simulink model "Simulation_GFM"  (R2022b)
settings: Solver=FixedStepAuto  StartTime=0.0  StopTime=4  FixedStep=1e-6  RelTol=1e-3
model workspace (MAT data in the model file):
  Fbase = 50
  Filter_Ind = 0.00435
  Fs = 10000
  Series1_L = 0.004
  Series2_L = 0.00035
  Shunt_C = 2.2e-06
  Snubber_C = inf
  Snubber_R = 100000
  Test_Interval = 3
  Ts = 0.0001
  VDCref = 48
undefined symbols (not defined in the file): DiscIntNeverNeededParam, Rdamp, Series1_C, Series2_R
libraries: spsThreePhaseSeriesRLCBranchLib x7, spsPWMGeneratorDCDCLib x3, spsVoltageMeasurementLib x3, spsabctodq0Lib x2, spsDCVoltageSourceLib x1, spsThreePhaseVIMeasurementLib x1, spsdq0toabcLib x1, spsUniversalBridgeLib x1, spspowerguiLib x1
settings Model: NumberOfSteps=10000  SnapshotBufferSize=10000  SnapshotInterval=10000  Creator=yanni  LastModifiedBy=yanni

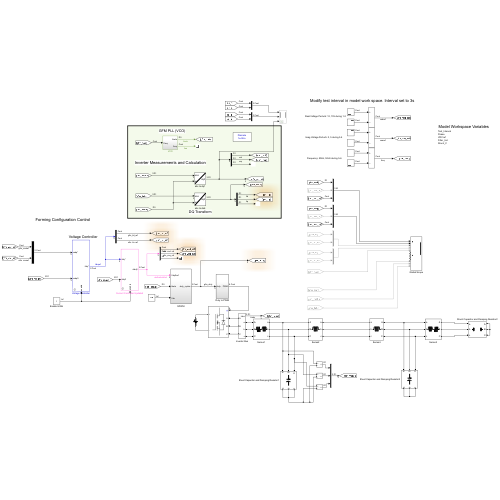
[thumbnail: Simulink's stored preview of the top-level diagram]
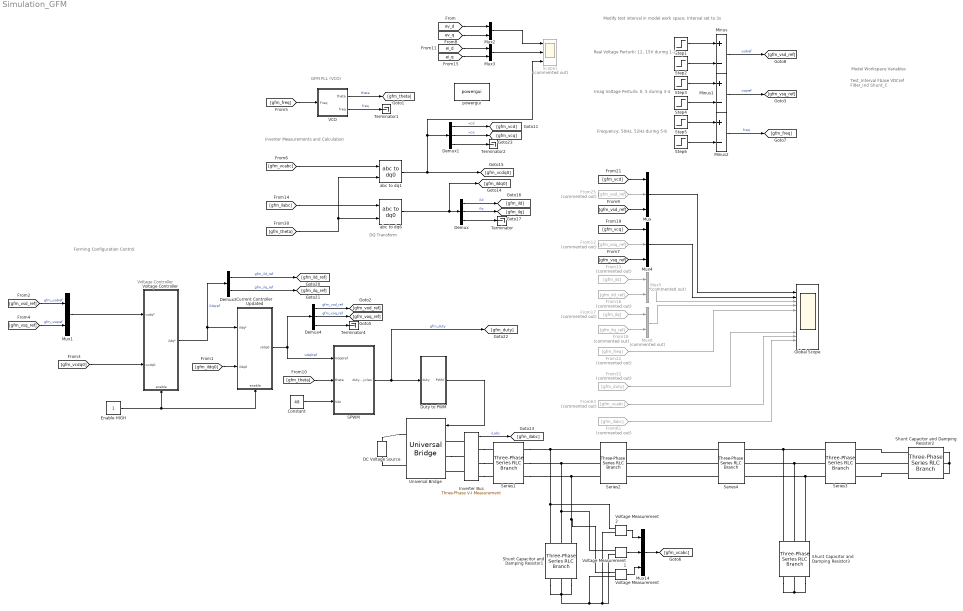
== system Simulation_GFM ==
  note: DQ Transform
  note: Forming Configuration Control
  note: Inverter Measurements and Calculation
  note: Voltage Controller
  note: Model Workspace Variables
  note: Real Voltage Perturb: 12, 15V during 1-2
  note: Imag Voltage Perturb: 0, 5 during 3-4
  note: Frequency: 50Hz, 52Hz during 5-6
  note: Test_Interval
      | Fbase
      | VDCref
      | Filter_Ind
      | Shunt_C
  note: Modify test interval in model work space. Interval set to 3s
  note: GFM PLL (VCO)
  Constant : Constant  Value=48
  Current Controller Updated : Subsystem  mask{Id_Proportional=1.22, Id_Integral=957}
      mask prompts: Id_Proportional "Kp"; Id_Integral "Ki"
      settings: PortSchema="{\"entries\":[{\"content\":{\"sides\":[{\"content\":{\"connectorIds\":[\"In1\",\"In2\"]},\"type\":\"ConnectorPlacement.EquallySpacedRectSide\",\"uuid\":\"134caf41-c34b-48d0-a71a-522329c40d8c\"},{\"content\":{\"connectorIds\":[\"Out1\"],\"side\":\"RIGHT\"},\"type\":\"ConnectorPlacement.EquallySpacedRectSide\",\"uuid\":\"de6d8359-09d9-4cb7-8990-bc4b6d48f18d\"},{\"content\":{\"connectorIds\":[],\"side\":\"TOP\"},\"type\":\"ConnectorPlacement.EquallySpacedRectSide\",\"uuid\":\"e2785d07-2ead-4d42-94ac-8025f550e46a\"},{\"content\":{\"connectorIds\":[\"In3\"],\"side\":\"BOTTOM\"},\"type\":\"ConnectorPlacement.EquallySpacedRectSide\",\"uuid\":\"a912a274-012c-4cba-911c-beb79bb7dc91\"}]},\"type\":\"ConnectorPlacement.EquallySpacedConnector\",\"uuid\":\"3c498838-bb9a-4b09-bf48-00f71cabf7b4\"}],\"packageUris\":[\"http://schema.mathworks.com/mf0/Connector/R2020b\"],\"version\":\"1.0\"}"
  DC Voltage Source : spsDCVoltageSourceLib/DC Voltage Source  Amplitude=48  Measurements=None
  Demux : Demux  Outputs=3
  Demux1 : Demux  Outputs=3
  Demux3 : Demux  Outputs=2
  Demux4 : Demux  Outputs=3
  Duty to PWM : Subsystem
  Enable HIGH : Constant
  From12 : From  Commented=on  GotoTag=gfm_voq_ref
      settings: CloseFcn=tagdialog Close
  From13 : From  Commented=on  GotoTag=gfm_ild
      settings: CloseFcn=tagdialog Close
  From16 : From  Commented=on  GotoTag=gfm_ild_ref
      settings: CloseFcn=tagdialog Close
  From17 : From  Commented=on  GotoTag=gfm_ilq
      settings: CloseFcn=tagdialog Close
  From18 : From  Commented=on  GotoTag=gfm_ilq_ref
      settings: CloseFcn=tagdialog Close
  From22 : From  Commented=on  GotoTag=gfm_freq
  From25 : From  Commented=on  GotoTag=gfm_vod_ref
      settings: CloseFcn=tagdialog Close
  From32 : From  Commented=on  GotoTag=gfm_duty
      settings: CloseFcn=tagdialog Close
  From61 : From  Commented=on  GotoTag=gfm_ilabc
      settings: CloseFcn=tagdialog Close
  From63 : From  Commented=on  GotoTag=gfm_vcabc
      settings: CloseFcn=tagdialog Close
  Global Scope : Scope  NumInputPorts=12
  Inverter Bus : spsThreePhaseVIMeasurementLib/Three-Phase V-I Measurement  VoltageMeasurement=no  SetLabelV=off  LabelV=Vabc  Vpu=off  VpuLL=off  CurrentMeasurement=yes  SetLabelI=off  LabelI=Iabc  Ipu=off  Pbase=100e6  Vbase=500e3  OutputType=Complex  PhasorSimulation=off  PSBequivalent=0
  Minus : Sum  Inputs=+-
  Minus1 : Sum  Inputs=+-
  Minus2 : Sum  Inputs=+-
  Mux : Mux  Inputs=3
  Mux1 : Mux  Inputs=2
  Mux14 : Mux  Inputs=3
  Mux2 : Mux  Inputs=2
  Mux3 : Mux  Inputs=2
  Mux4 : Mux  Inputs=3
  Mux5 : Mux  Commented=on  Inputs=2
  Mux6 : Mux  Commented=on  Inputs=2
  SPWM : Subsystem
  Scope1 : Scope  Commented=on  NumInputPorts=3
  Series1 : spsThreePhaseSeriesRLCBranchLib/Three-Phase Series RLC Branch  LConnTagsString=A|B|C  RConnTagsString=A|B|C  BranchType=RL  Resistance=0.35  Inductance=Series1_L  Capacitance=Series1_C  Measurements=None
  Series2 : spsThreePhaseSeriesRLCBranchLib/Three-Phase Series RLC Branch  LConnTagsString=A|B|C  RConnTagsString=A|B|C  BranchType=L  Resistance=Series2_R  Inductance=Series2_L  Capacitance=1e-6  Measurements=None
  Series3 : spsThreePhaseSeriesRLCBranchLib/Three-Phase Series RLC Branch  LConnTagsString=A|B|C  RConnTagsString=A|B|C  BranchType=RL  Resistance=0.35  Inductance=Series1_L  Capacitance=Series1_C  Measurements=None
  Series4 : spsThreePhaseSeriesRLCBranchLib/Three-Phase Series RLC Branch  LConnTagsString=A|B|C  RConnTagsString=A|B|C  BranchType=L  Resistance=Series2_L  Inductance=Series2_L  Capacitance=1e-6  Measurements=None
  Shunt Capacitor and Damping Resistor1 : spsThreePhaseSeriesRLCBranchLib/Three-Phase Series RLC Branch  LConnTagsString=A|B|C  RConnTagsString=A|B|C  BranchType=C  Resistance=Rdamp  Inductance=1e-3  Capacitance=2.2e-6  Measurements=None
  Shunt Capacitor and Damping Resistor2 : spsThreePhaseSeriesRLCBranchLib/Three-Phase Series RLC Branch  LConnTagsString=A|B|C  RConnTagsString=A|B|C  BranchType=Open circuit  Resistance=20  Inductance=1e-3  Capacitance=Shunt_C  Measurements=None
  Shunt Capacitor and Damping Resistor3 : spsThreePhaseSeriesRLCBranchLib/Three-Phase Series RLC Branch  LConnTagsString=A|B|C  RConnTagsString=A|B|C  BranchType=C  Resistance=Rdamp  Inductance=1e-3  Capacitance=2.2e-6  Measurements=None
  Step1 : Step  Time=Test_Interval*1  Before=12  After=15
  Step2 : Step  Time=Test_Interval*2  After=3
  Step3 : Step  Time=Test_Interval*3  After=5
  Step4 : Step  Time=Test_Interval*4  After=5
  Step5 : Step  Time=Test_Interval*5  Before=50  After=52  SampleTime=0
  Step6 : Step  Time=Test_Interval*6  After=2
  Terminator{,1..2,4} (4 alike) : Terminator
  Universal Bridge : spsUniversalBridgeLib/Universal Bridge  Arms=3  SnubberResistance=Snubber_R  SnubberCapacitance=Snubber_C  Device=MOSFET / Diodes  Ron=1e-3  Lon=0  ForwardVoltages="[  0  0  ]"  ForwardVoltage=0  GTOparameters=[ 10e-6 , 20e-6 ]  IGBTparameters=[ 1e-6 , 2e-6 ]  Measurements=None  Measurements_2=None  converterType=Rectifier
  VCO : Subsystem
  Voltage Controller : Subsystem  mask{Id_Proportional=0.028, Id_Integral=8.8685}
      mask prompts: Id_Proportional "Kp"; Id_Integral "Ki"
      settings: PortSchema="{\"entries\":[{\"content\":{\"sides\":[{\"content\":{\"connectorIds\":[\"In1\",\"In2\"]},\"type\":\"ConnectorPlacement.EquallySpacedRectSide\",\"uuid\":\"134caf41-c34b-48d0-a71a-522329c40d8c\"},{\"content\":{\"connectorIds\":[\"Out1\"],\"side\":\"RIGHT\"},\"type\":\"ConnectorPlacement.EquallySpacedRectSide\",\"uuid\":\"de6d8359-09d9-4cb7-8990-bc4b6d48f18d\"},{\"content\":{\"connectorIds\":[],\"side\":\"TOP\"},\"type\":\"ConnectorPlacement.EquallySpacedRectSide\",\"uuid\":\"e2785d07-2ead-4d42-94ac-8025f550e46a\"},{\"content\":{\"connectorIds\":[\"In3\"],\"side\":\"BOTTOM\"},\"type\":\"ConnectorPlacement.EquallySpacedRectSide\",\"uuid\":\"a912a274-012c-4cba-911c-beb79bb7dc91\"}]},\"type\":\"ConnectorPlacement.EquallySpacedConnector\",\"uuid\":\"3c498838-bb9a-4b09-bf48-00f71cabf7b4\"}],\"packageUris\":[\"http://schema.mathworks.com/mf0/Connector/R2020b\"],\"version\":\"1.0\"}"
  Voltage Measurement : spsVoltageMeasurementLib/Voltage Measurement  PhasorSimulation=off  OutputType=Complex  PSBequivalent=0
  Voltage Measurement1 : spsVoltageMeasurementLib/Voltage Measurement  PhasorSimulation=off  OutputType=Complex  PSBequivalent=0
  Voltage Measurement2 : spsVoltageMeasurementLib/Voltage Measurement  PhasorSimulation=off  OutputType=Complex  PSBequivalent=0
  abc to dq1 : spsabctodq0Lib/abc to dq0  Alignment=90 degrees behind phase A axis
  abc to dq6 : spsabctodq0Lib/abc to dq0  Alignment=90 degrees behind phase A axis
  powergui : spspowerguiLib/powergui  Priority=1  SimulationMode=Discrete  SampleTime=1e-6  frequency=60  Iterations=50  frequencyindice=0  Pbase=100e6  ErrMax=1e-4  UnitsV=kV  UnitsW=MW  buscounter=0  FunctionMessages=off  echomessages=off  EnableUseOfTLC=off  CurrentSourceSwitches=off  DisableSnubberDevices=off  DisableRonSwitches=off  DisableVfSwitches=off  DisplayEquations=off  AutomaticDiscreteSolvers=off  SolverType=Tustin/Backward Euler (TBE)  Interpol=off  ExternalGateDelay=off  methode=off  Ts=100  x0status=blocks  SPID=on  SwTol=0  HookPort=off  NonlinearTolerance=1e-4  nMaxIteration=100  ContinueOnMaxIteration=off  RestoreLinks=warning  ResistiveCurrentMeasurement=off  Frange=[0:2:500]  Ylog=off  Xlog=on  ShowGrid=off  save=off  variable=ZData  structure=0  ZoomFFT=off  StartTime=0.0  cycles=1  DisplayStyle=1  fundamental=60  FreqAxis=off  MaxFrequency=1000  frequencyindicesteady=1  RmsSteady=1  display=off
  wires:
  abc to dq1/1 -> Demux1/1, Scope1/3, [gfm_vcdq0]
  Current Controller Updated/1(vtdq0) -> SPWM/1(Vdq0ref), Demux4/1  "vdq0ref"
  abc to dq6/1 -> [gfm_ildq0], Demux/1
  [gfm_theta] -> SPWM/2(theta)
  Enable HIGH/1 -> Current Controller Updated/3(enable), Voltage Controller/3(enable)
  Mux1/1 -> Voltage Controller/1(vsdq*)
  Inverter Bus/1 -> [gfm_ilabc]  "iLabc"
  Demux/2 -> [gfm_ilq]  "ilq"
  Demux/1 -> [gfm_ild]  "ild"
  Demux/3 -> Terminator/1
  Demux3/2 -> [gfm_ilq_ref]  "gfm_ilq_ref"
  Demux3/1 -> [gfm_ild_ref]  "gfm_ild_ref"
  Demux4/2 -> [gfm_voq_ref]  "gfm_voq_ref"
  Demux4/1 -> [gfm_vod_ref]  "gfm_vod_ref"
  Demux4/3 -> Terminator4/1
  [gfm_theta] -> abc to dq1/2, abc to dq6/2
  Voltage Controller/1(ildq*) -> Demux3/1, Current Controller Updated/1(ildq*)  "ildqref"
  [gfm_ilabc] -> abc to dq6/1
  Duty to PWM/1(PWM) -> Universal Bridge/1
  SPWM/1(duty_cycles) -> Duty to PWM/1(duty), [gfm_duty]  "gfm_duty"
  From25/1 -> Mux/2
  From17/1 -> Mux6/1
  Mux/1 -> Global Scope/1
  From63/1 -> Global Scope/11
  From32/1 -> Global Scope/10
  From12/1 -> Mux4/2
  Mux4/1 -> Global Scope/2
  [gfm_vcd] -> Mux/1
  Mux5/1 -> Global Scope/3
  From61/1 -> Global Scope/12
  Mux6/1 -> Global Scope/4
  From16/1 -> Mux5/2
  From13/1 -> Mux5/1
  From18/1 -> Mux6/2
  [gfm_vcq] -> Mux4/1
  [gfm_vsd_ref] -> Mux/3
  [gfm_vsq_ref] -> Mux4/3
  Demux1/2 -> [gfm_vcq]  "vcq"
  Demux1/1 -> [gfm_vcd]  "vcd"
  Demux1/3 -> Terminator2/1
  [gfm_vcabc] -> abc to dq1/1
  [gfm_vcdq0] -> Voltage Controller/2(vcdq0)
  Constant/1 -> SPWM/3(Vdc)
  Minus/1 -> [gfm_vsd_ref]  "vsdref"
  Step3/1 -> Minus1/1
  Step2/1 -> Minus/2
  Minus1/1 -> [gfm_vsq_ref]  "vsqref"
  Step5/1 -> Minus2/1
  Step4/1 -> Minus1/2
  Step1/1 -> Minus/1
  Minus2/1 -> [gfm_freq]  "freq"
  Step6/1 -> Minus2/2
  From22/1 -> Global Scope/5
  [gfm_ildq0] -> Current Controller Updated/2(ildq0)
  [gfm_vsd_ref] -> Mux1/1  "gfm_vsdref"
  [gfm_vsq_ref] -> Mux1/2  "gfm_vsqref"
  VCO/1(theta) -> [gfm_theta]  "theta"
  VCO/2(freq) -> Terminator1/1  "freq"
  [gfm_freq] -> VCO/1(Freq)
  Mux14/1 -> [gfm_vcabc]
  Voltage Measurement/1 -> Mux14/3
  Voltage Measurement1/1 -> Mux14/2
  Voltage Measurement2/1 -> Mux14/1
  Mux3/1 -> Scope1/2
  Mux2/1 -> Scope1/1
  [ev_d] -> Mux2/1
  [ev_q] -> Mux2/2
  [ei_d] -> Mux3/1
  [ei_q] -> Mux3/2
  connections:
  DC Voltage Source/LConn1 -- Universal Bridge/RConn2
  Universal Bridge/RConn1 -- DC Voltage Source/RConn1
  Shunt Capacitor and Damping Resistor1/LConn2 -- Series2/LConn2 -- Series1/RConn2 -- Voltage Measurement1/LConn1
  Voltage Measurement/LConn1 -- Series2/LConn3 -- Series1/RConn3 -- Shunt Capacitor and Damping Resistor1/LConn3
  Voltage Measurement2/LConn1 -- Series2/LConn1 -- Series1/RConn1 -- Shunt Capacitor and Damping Resistor1/LConn1
  Inverter Bus/RConn2 -- Series1/LConn2
  Inverter Bus/RConn1 -- Series1/LConn1
  Inverter Bus/RConn3 -- Series1/LConn3
  Inverter Bus/LConn1 -- Universal Bridge/LConn1
  Universal Bridge/LConn2 -- Inverter Bus/LConn2
  Inverter Bus/LConn3 -- Universal Bridge/LConn3
  Shunt Capacitor and Damping Resistor2/LConn1 -- Shunt Capacitor and Damping Resistor2/LConn2 -- Shunt Capacitor and Damping Resistor2/LConn3
  Shunt Capacitor and Damping Resistor1/RConn2 -- Voltage Measurement/LConn2 -- Voltage Measurement2/LConn2 -- Voltage Measurement1/LConn2 -- Shunt Capacitor and Damping Resistor1/RConn1 -- Shunt Capacitor and Damping Resistor1/RConn3
  Shunt Capacitor and Damping Resistor3/RConn2 -- Shunt Capacitor and Damping Resistor3/RConn3 -- Shunt Capacitor and Damping Resistor3/RConn1
  Shunt Capacitor and Damping Resistor3/LConn2 -- Series3/RConn2 -- Series4/LConn2
  Shunt Capacitor and Damping Resistor3/LConn3 -- Series3/RConn3 -- Series4/LConn3
  Shunt Capacitor and Damping Resistor3/LConn1 -- Series3/RConn1 -- Series4/LConn1
  Shunt Capacitor and Damping Resistor2/RConn1 -- Series3/LConn1
  Shunt Capacitor and Damping Resistor2/RConn3 -- Series3/LConn3
  Shunt Capacitor and Damping Resistor2/RConn2 -- Series3/LConn2
  Series4/RConn1 -- Series2/RConn1
  Series4/RConn2 -- Series2/RConn2
  Series4/RConn3 -- Series2/RConn3

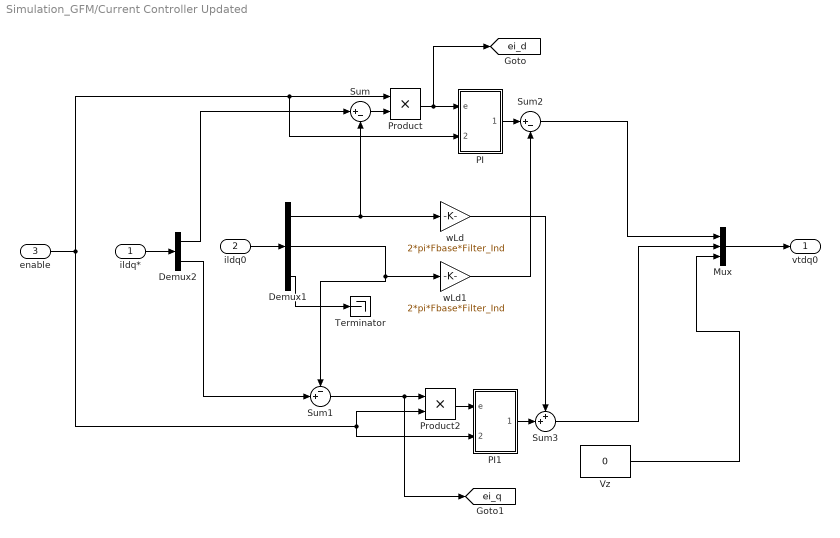
== system Simulation_GFM/Current Controller Updated ==
  ildq* : Inport
  ildq0 : Inport  Port=2
  enable : Inport  Port=3
  Demux1 : Demux  Outputs=3
  Demux2 : Demux  Outputs=2
  Mux : Mux  Inputs=3
  PI : Subsystem
  PI1 : Subsystem
  Product : Product  RndMeth=Zero
  Product2 : Product  RndMeth=Zero
  Sum : Sum  Inputs=|+-
  Sum1 : Sum  Inputs=-+|
  Sum2 : Sum  Inputs=|+-
  Sum3 : Sum  Inputs=++|
  Terminator : Terminator
  Vz : Constant  Value=0
  wLd : Gain  Gain=2*pi*Fbase*Filter_Ind
  wLd1 : Gain  Gain=2*pi*Fbase*Filter_Ind
  vtdq0 : Outport
  tag scope: ei_d=global, ei_q=global
  wires:
  Sum2/1 -> Mux/1
  Sum3/1 -> Mux/2
  ildq0/1 -> Demux1/1
  Mux/1 -> vtdq0/1
  Demux1/3 -> Terminator/1
  ildq*/1 -> Demux2/1
  Demux2/1 -> Sum/1
  Demux2/2 -> Sum1/2
  PI/1(Out) -> Sum2/1
  wLd/1 -> Sum3/1
  wLd1/1 -> Sum2/2
  PI1/1(Out) -> Sum3/2
  Demux1/2 -> Sum1/1, wLd1/1
  Demux1/1 -> wLd/1, Sum/2
  Product2/1 -> PI1/1(e)
  Sum/1 -> Product/2
  enable/1 -> Product/1, PI/2(RST), PI1/2(RST), Product2/2
  Vz/1 -> Mux/3
  Sum1/1 -> [ei_q], Product2/1
  Product/1 -> [ei_d], PI/1(e)

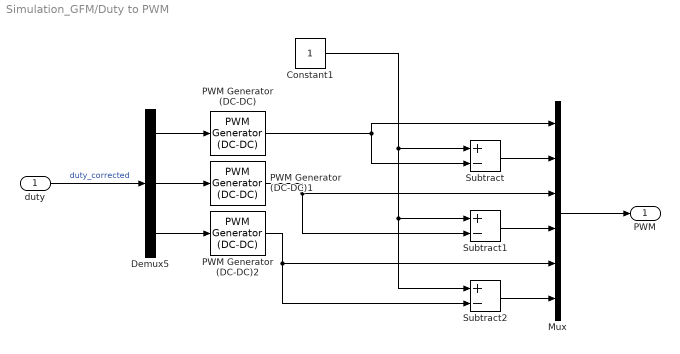
== system Simulation_GFM/Duty to PWM ==
  duty : Inport
  Constant1 : Constant
  Demux5 : Demux  Outputs=3
  Mux : Mux  Inputs=6
  PWM Generator (DC-DC) : spsPWMGeneratorDCDCLib/PWM Generator (DC-DC)  Fsw=Fs  Ts=0
  PWM Generator (DC-DC)1 : spsPWMGeneratorDCDCLib/PWM Generator (DC-DC)  Fsw=Fs  Ts=0
  PWM Generator (DC-DC)2 : spsPWMGeneratorDCDCLib/PWM Generator (DC-DC)  Fsw=Fs  Ts=0
  Subtract : Sum  Inputs=+-
  Subtract1 : Sum  Inputs=+-
  Subtract2 : Sum  Inputs=+-
  PWM : Outport
  wires:
  PWM Generator (DC-DC)1/1 -> Subtract1/2, Mux/3
  Demux5/2 -> PWM Generator (DC-DC)1/1
  Demux5/1 -> PWM Generator (DC-DC)/1
  Demux5/3 -> PWM Generator (DC-DC)2/1
  PWM Generator (DC-DC)2/1 -> Subtract2/2, Mux/5
  duty/1 -> Demux5/1  "duty_corrected"
  Subtract1/1 -> Mux/4
  Subtract2/1 -> Mux/6
  PWM Generator (DC-DC)/1 -> Mux/1, Subtract/2
  Constant1/1 -> Subtract2/1, Subtract1/1, Subtract/1
  Subtract/1 -> Mux/2
  Mux/1 -> PWM/1

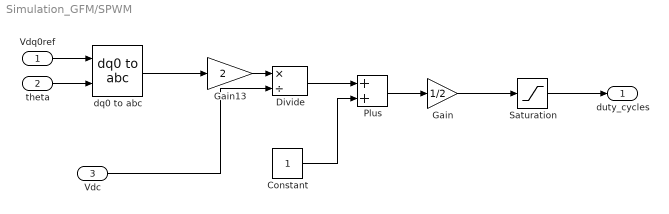
== system Simulation_GFM/SPWM ==
  Vdq0ref : Inport
  theta : Inport  Port=2
  Vdc : Inport  Port=3
  Constant : Constant
  Divide : Product  Inputs=*/
  Gain : Gain  Gain=1/2
  Gain13 : Gain  Gain=2
  Plus : Sum
  Saturation : Saturate  UpperLimit=0.9  LowerLimit=0.1
  dq0 to abc : spsdq0toabcLib/dq0 to abc  Alignment=90 degrees behind phase A axis
  duty_cycles : Outport
  wires:
  Vdq0ref/1 -> dq0 to abc/1
  Gain/1 -> Saturation/1
  theta/1 -> dq0 to abc/2
  Constant/1 -> Plus/2
  Plus/1 -> Gain/1
  Saturation/1 -> duty_cycles/1
  dq0 to abc/1 -> Gain13/1
  Gain13/1 -> Divide/1
  Vdc/1 -> Divide/2
  Divide/1 -> Plus/1

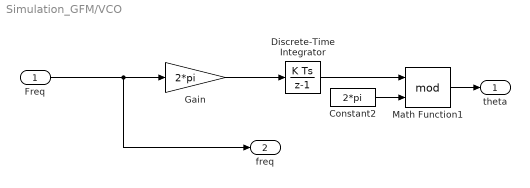
== system Simulation_GFM/VCO ==
  Freq : Inport
  Constant2 : Constant  Value=2*pi
  Discrete-Time Integrator : DiscreteIntegrator  SampleTime=Ts  ICPrevOutput=DiscIntNeverNeededParam  ICPrevScaledInput=DiscIntNeverNeededParam
  Gain : Gain  Gain=2*pi
  Math Function1 : Math  Operator=mod  SignedPower=on
  theta : Outport
  freq : Outport  Port=2
  wires:
  Constant2/1 -> Math Function1/2
  Discrete-Time Integrator/1 -> Math Function1/1
  Math Function1/1 -> theta/1
  Freq/1 -> Gain/1, freq/1
  Gain/1 -> Discrete-Time Integrator/1

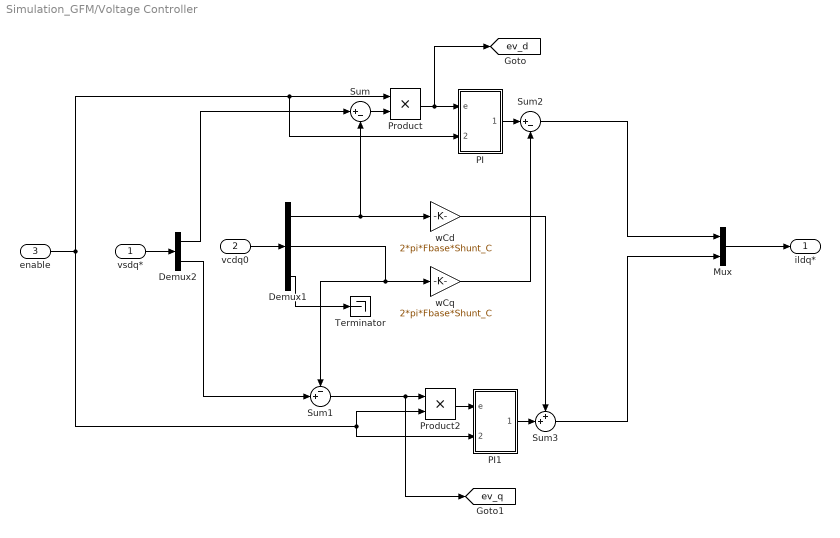
== system Simulation_GFM/Voltage Controller ==
  vsdq* : Inport
  vcdq0 : Inport  Port=2
  enable : Inport  Port=3
  Demux1 : Demux  Outputs=3
  Demux2 : Demux  Outputs=2
  Mux : Mux  Inputs=2
  PI : Subsystem
  PI1 : Subsystem
  Product : Product  RndMeth=Zero
  Product2 : Product  RndMeth=Zero
  Sum : Sum  Inputs=|+-
  Sum1 : Sum  Inputs=-+|
  Sum2 : Sum  Inputs=|+-
  Sum3 : Sum  Inputs=++|
  Terminator : Terminator
  wCd : Gain  Gain=2*pi*Fbase*Shunt_C
  wCq : Gain  Gain=2*pi*Fbase*Shunt_C
  ildq* : Outport
  tag scope: ev_d=global, ev_q=global
  wires:
  Sum2/1 -> Mux/1
  Sum3/1 -> Mux/2
  vcdq0/1 -> Demux1/1
  Mux/1 -> ildq*/1
  Demux1/3 -> Terminator/1
  vsdq*/1 -> Demux2/1
  Demux2/1 -> Sum/1
  Demux2/2 -> Sum1/2
  Product/1 -> [ev_d], PI/1(e)
  Sum1/1 -> [ev_q], Product2/1
  PI/1(Out) -> Sum2/1
  wCd/1 -> Sum3/1
  wCq/1 -> Sum2/2
  PI1/1(Out) -> Sum3/2
  Demux1/2 -> Sum1/1, wCq/1
  Demux1/1 -> wCd/1, Sum/2
  Product2/1 -> PI1/1(e)
  Sum/1 -> Product/2
  enable/1 -> Product/1, PI/2(RST), PI1/2(RST), Product2/2

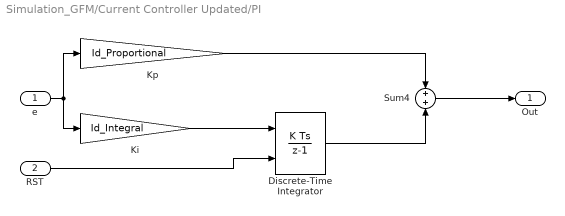
== system Simulation_GFM/Current Controller Updated/PI ==
  e : Inport
  RST : Inport  Port=2
  Discrete-Time Integrator : DiscreteIntegrator  gainval=1  ExternalReset=either  SampleTime=Ts  LimitOutput=on  UpperSaturationLimit=20000  LowerSaturationLimit=-20000  ICPrevOutput=DiscIntNeverNeededParam  ICPrevScaledInput=DiscIntNeverNeededParam
  Ki : Gain  Gain=Id_Integral  SaturateOnIntegerOverflow=on  OutDataTypeStr=Inherit: Same as input  ParamDataTypeStr=Inherit: Same as input
  Kp : Gain  Gain=Id_Proportional  SaturateOnIntegerOverflow=on  OutDataTypeStr=Inherit: Same as input  ParamDataTypeStr=Inherit: Same as input
  Sum4 : Sum  SaturateOnIntegerOverflow=on
  Out : Outport
  wires:
  Ki/1 -> Discrete-Time Integrator/1
  Kp/1 -> Sum4/1
  e/1 -> Ki/1, Kp/1
  Discrete-Time Integrator/1 -> Sum4/2
  Sum4/1 -> Out/1
  RST/1 -> Discrete-Time Integrator/2

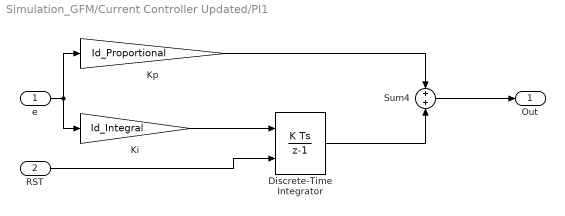
== system Simulation_GFM/Current Controller Updated/PI1 ==
  e : Inport
  RST : Inport  Port=2
  Discrete-Time Integrator : DiscreteIntegrator  gainval=1  ExternalReset=either  SampleTime=Ts  LimitOutput=on  UpperSaturationLimit=20000  LowerSaturationLimit=-20000  ICPrevOutput=DiscIntNeverNeededParam  ICPrevScaledInput=DiscIntNeverNeededParam
  Ki : Gain  Gain=Id_Integral  SaturateOnIntegerOverflow=on  OutDataTypeStr=Inherit: Same as input  ParamDataTypeStr=Inherit: Same as input
  Kp : Gain  Gain=Id_Proportional  SaturateOnIntegerOverflow=on  OutDataTypeStr=Inherit: Same as input  ParamDataTypeStr=Inherit: Same as input
  Sum4 : Sum  SaturateOnIntegerOverflow=on
  Out : Outport
  wires:
  Ki/1 -> Discrete-Time Integrator/1
  Kp/1 -> Sum4/1
  e/1 -> Ki/1, Kp/1
  Discrete-Time Integrator/1 -> Sum4/2
  Sum4/1 -> Out/1
  RST/1 -> Discrete-Time Integrator/2

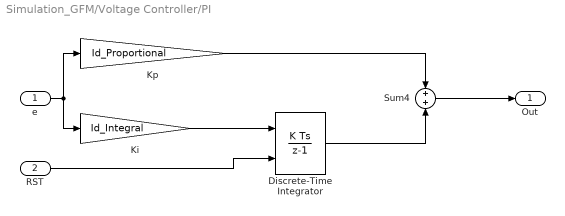
== system Simulation_GFM/Voltage Controller/PI ==
  e : Inport
  RST : Inport  Port=2
  Discrete-Time Integrator : DiscreteIntegrator  gainval=1  ExternalReset=either  SampleTime=Ts  LimitOutput=on  UpperSaturationLimit=2000  LowerSaturationLimit=-2000  ICPrevOutput=DiscIntNeverNeededParam  ICPrevScaledInput=DiscIntNeverNeededParam
  Ki : Gain  Gain=Id_Integral  SaturateOnIntegerOverflow=on  OutDataTypeStr=Inherit: Same as input  ParamDataTypeStr=Inherit: Same as input
  Kp : Gain  Gain=Id_Proportional  SaturateOnIntegerOverflow=on  OutDataTypeStr=Inherit: Same as input  ParamDataTypeStr=Inherit: Same as input
  Sum4 : Sum  SaturateOnIntegerOverflow=on
  Out : Outport
  wires:
  Ki/1 -> Discrete-Time Integrator/1
  Kp/1 -> Sum4/1
  e/1 -> Ki/1, Kp/1
  Discrete-Time Integrator/1 -> Sum4/2
  Sum4/1 -> Out/1
  RST/1 -> Discrete-Time Integrator/2

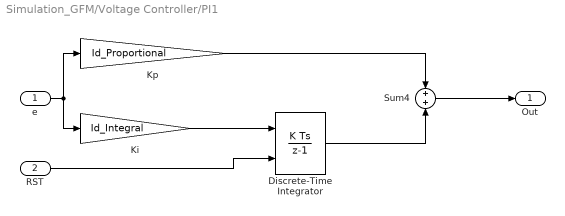
== system Simulation_GFM/Voltage Controller/PI1 ==
  e : Inport
  RST : Inport  Port=2
  Discrete-Time Integrator : DiscreteIntegrator  gainval=1  ExternalReset=either  SampleTime=Ts  LimitOutput=on  UpperSaturationLimit=2000  LowerSaturationLimit=-2000  ICPrevOutput=DiscIntNeverNeededParam  ICPrevScaledInput=DiscIntNeverNeededParam
  Ki : Gain  Gain=Id_Integral  SaturateOnIntegerOverflow=on  OutDataTypeStr=Inherit: Same as input  ParamDataTypeStr=Inherit: Same as input
  Kp : Gain  Gain=Id_Proportional  SaturateOnIntegerOverflow=on  OutDataTypeStr=Inherit: Same as input  ParamDataTypeStr=Inherit: Same as input
  Sum4 : Sum  SaturateOnIntegerOverflow=on
  Out : Outport
  wires:
  Ki/1 -> Discrete-Time Integrator/1
  Kp/1 -> Sum4/1
  e/1 -> Ki/1, Kp/1
  Discrete-Time Integrator/1 -> Sum4/2
  Sum4/1 -> Out/1
  RST/1 -> Discrete-Time Integrator/2
